simulink model "Control_Robot"  (R2018a)
settings: Solver=FixedStepAuto  StartTime=0.0  StopTime=10.0  FixedStep=0.01  RelTol=1e-3
undefined symbols (not defined in the file or in its folder): sigbuilder_block
libraries: simulink x2
settings Model: Creator=Amin  LastModifiedBy=Amin

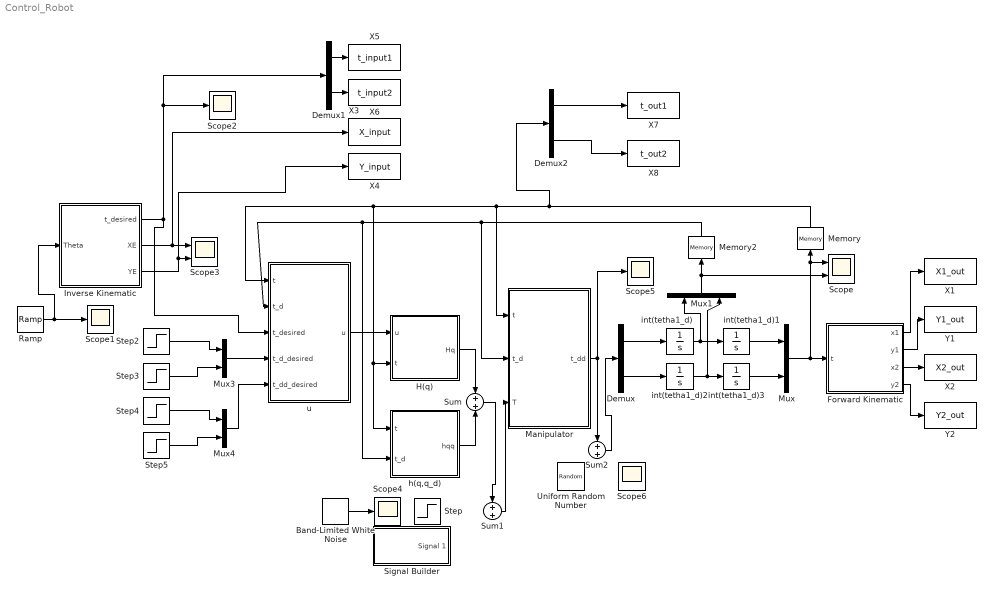
== system Control_Robot ==
   int(tetha1_d){,1..3} (4 alike) : Integrator
  Band-Limited White Noise : simulink/Sources/Band-Limited White Noise  Cov=[0.05]  Ts=0.1  seed=[23341]
  Demux : Demux  Outputs=2
  Demux1 : Demux  Outputs=2
  Demux2 : Demux  Outputs=2
  Forward Kinematic : MATLAB Function  TreatAsAtomicUnit=on
  H(q) : MATLAB Function  TreatAsAtomicUnit=on
  Inverse Kinematic : MATLAB Function  TreatAsAtomicUnit=on
  Manipulator : MATLAB Function  TreatAsAtomicUnit=on
  Memory : Memory  InitialCondition=[0 0]
  Memory2 : Memory  InitialCondition=[0 0]
  Mux{,1,3..4} (4 alike) : Mux  Inputs=2
  Ramp : simulink/Sources/Ramp  slope=1  start=1  InitialOutput=0
  Scope : Scope  NumInputPorts=2
  Scope{1..2,4..6} (5 alike) : Scope
  Scope3 : Scope  NumInputPorts=2
  Signal Builder : Subsystem  Tag=STV Subsys  LoadFcn=sigbuilder_block('load');  StartFcn=sigbuilder_block('start');  StopFcn=sigbuilder_block('stop');  ClipboardFcn=sigbuilder_block('clipboard');  mask(Sigbuilder block){tuvar=[0:10]}
      mask help: Simulink:masks:SigbuilderBlock_MD
      mask init:
      | if ~strcmp(get_param(bdroot(gcbh),'SimulationStatus'),'stopped') tuvar = sigbuilder_block('maskInit'); end
      settings: CopyFcn=sigbuilder_block('copy');  DeleteFcn=sigbuilder_block('delete');  ModelCloseFcn=sigbuilder_block('modelClose');  PreSaveFcn=sigbuilder_block('preSave');  PauseFcn=sigbuilder_block('pause');  ContinueFcn=sigbuilder_block('continue');  NameChangeFcn=sigbuilder_block('namechange');  OpenFcn=sigbuilder_block('open',[93 131.25 550.5 359.25 ]);  CloseFcn=sigbuilder_block('close');
      mask Display: plot(0, 0, 100, 100,[2, 2, 32, 32, 2], [68, 8, 8, 68, 68],[32, 2], [38, 38], [32, 19, 2],[53, 60, 44], [32, 17, 17, 2],[16, 16, 31, 31]);txt = getActiveGroup(gcbh);text(2, 100, txt,'verticalAlignment', 'top');
  Step : Step  After=6  SampleTime=0
  Step2 : Step  Before=0.01  After=0.01  SampleTime=0
  Step3 : Step  Before=0.01  After=0.01  SampleTime=0
  Step4 : Step  Before=0.001  After=0.001  SampleTime=0
  Step5 : Step  Before=0.001  After=0.001  SampleTime=0
  Sum : Sum  Inputs=+|+
  Sum1 : Sum  Inputs=+|+
  Sum2 : Sum  Inputs=+|+
  Uniform Random Number : UniformRandomNumber  Minimum=-3  Maximum=3  SampleTime=0.1
  X1 : ToWorkspace  VariableName=X1_out  SaveFormat=Structure With Time  SampleTime=-1
  X2 : ToWorkspace  VariableName=X2_out  SaveFormat=Structure With Time  SampleTime=-1
  X3 : ToWorkspace  VariableName=X_input  SaveFormat=Structure With Time  SampleTime=-1
  X4 : ToWorkspace  VariableName=Y_input  SaveFormat=Structure With Time  SampleTime=-1
  X5 : ToWorkspace  VariableName=t_input1  SaveFormat=Structure With Time  SampleTime=-1
  X6 : ToWorkspace  VariableName=t_input2  SaveFormat=Structure With Time  SampleTime=-1
  X7 : ToWorkspace  VariableName=t_out1  SaveFormat=Structure With Time  SampleTime=-1
  X8 : ToWorkspace  VariableName=t_out2  SaveFormat=Structure With Time  SampleTime=-1
  Y1 : ToWorkspace  VariableName=Y1_out  SaveFormat=Structure With Time  SampleTime=-1
  Y2 : ToWorkspace  VariableName=Y2_out  SaveFormat=Structure With Time  SampleTime=-1
  h(q,q_d) : MATLAB Function  TreatAsAtomicUnit=on
  u : MATLAB Function  TreatAsAtomicUnit=on
  wires:
  " int(tetha1_d)"/1 -> Mux1/1, " int(tetha1_d)1"/1
  " int(tetha1_d)2"/1 -> Mux1/2, " int(tetha1_d)3"/1
  Demux/1 -> " int(tetha1_d)"/1
  Demux/2 -> " int(tetha1_d)2"/1
  " int(tetha1_d)3"/1 -> Mux/2
  Mux/1 -> Scope/1, Memory/1, Forward Kinematic/1(t)
  Mux1/1 -> Scope/2, Memory2/1
  H(q)/1(Hq) -> Sum/1
  h(q,q_d)/1(hqq) -> Sum/2
  Memory2/1 -> Manipulator/2(t_d), u/2(t_d), h(q,q_d)/2(t_d)
  Memory/1 -> Demux2/1, u/1(t), h(q,q_d)/1(t), H(q)/2(t), Manipulator/1(t)
  u/1(u) -> H(q)/1(u)
  Forward Kinematic/1(x1) -> X1/1
  Forward Kinematic/2(y1) -> Y1/1
  Forward Kinematic/3(x2) -> X2/1
  Forward Kinematic/4(y2) -> Y2/1
  Step3/1 -> Mux3/2
  Step2/1 -> Mux3/1
  Step4/1 -> Mux4/1
  Step5/1 -> Mux4/2
  Mux4/1 -> u/5(t_dd_desired)
  Inverse Kinematic/1(t_desired) -> Demux1/1, Scope2/1, u/3(t_desired)
  Inverse Kinematic/2(XE) -> X3/1, Scope3/1
  Inverse Kinematic/3(YE) -> X4/1, Scope3/2
  Demux1/1 -> X5/1
  Demux1/2 -> X6/1
  Demux2/1 -> X7/1
  Demux2/2 -> X8/1
  Ramp/1 -> Scope1/1, Inverse Kinematic/1(Theta)
  Mux3/1 -> u/4(t_d_desired)
  " int(tetha1_d)1"/1 -> Mux/1
  Band-Limited White Noise/1 -> Scope4/1
  Manipulator/1(t_dd) -> Scope5/1, Sum2/1
  Sum2/1 -> Demux/1
  Sum/1 -> Sum1/1
  Sum1/1 -> Manipulator/3(T)

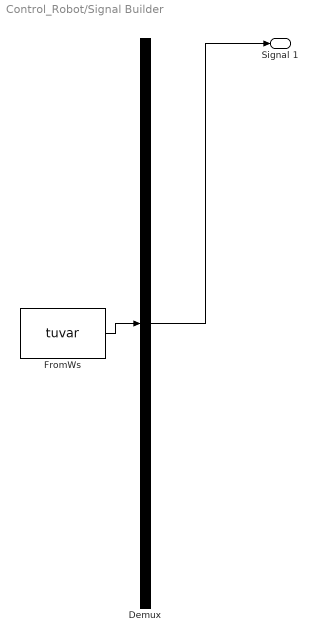
== system Control_Robot/Signal Builder ==
  Demux : Demux  Tag=STV Demux  Outputs=1
  FromWs : FromWorkspace  Tag=STV FromWs  VariableName=tuvar  SampleTime=0
      SigBuilderData=|
      | common.afterFinalStr = 'Extrapolate'
      | common.sampleTime = 0
      | dataSet.timeRange = [0 10]
      | dataSet.name = 'Group 1'
      | sbobj.Groups.Name = 'Group 1'
      | sbobj.Groups.Signals.Name = 'Signal 1'
      | sbobj.Groups.Signals.XData = [0 2.98 3 3 7 7 10]
      | sbobj.Groups.Signals.YData = [0 0 8 10 10 0 0]
  Signal 1 : Outport  Tag=STV Outport
  wires:
  Demux/1 -> Signal 1/1
  FromWs/1 -> Demux/1

== matlab function Control_Robot/H(q) ==
  data: u input; Hq output; t input
function Hq = fcn(u, t)
m1 = 1;
m2 = 1;
l1 = 1;
lc1 = 0.5;
l2 = 1;
lc2 = 0.5;
g = 9.81;

H11 = m1*lc1^2 + l1 + m2*(l1^2+lc2^2+2*l1*lc2*cos(t(2)))+l2;
H22 = m2*lc2^2 + l2;
H12 = m2*l1*lc2*cos(t(2)) + m2*lc2^2 + l2;
H21 = m2*l1*lc2*cos(t(2)) + m2*lc2^2 + l2;

H = [H11 H12; H21 H22];

Hq = H*u;

== matlab function Control_Robot/Manipulator ==
  data: t input; t_dd output; t_d input; T input
function t_dd = fcn(t, t_d, T)
m1 = 1;
m2 = 1;
l1 = 1;
lc1 = 0.5;
l2 = 1;
lc2 = 0.5;
g = 9.81;
H11 = m1*lc1^2 + l1 + m2*(l1^2+lc2^2+2*l1*lc2*cos(t(2)))+l2;
H22 = m2*lc2^2 + l2;
H12 = m2*l1*lc2*cos(t(2)) + m2*lc2^2 + l2;
H21 = m2*l1*lc2*cos(t(2)) + m2*lc2^2 + l2;
H = [H11 H12; H21 H22];
h = m2*l1*lc2*sin(t(2));
g1 = m1*lc1*g*cos(t(1)) + m2*g*(lc2*cos(t(1)+t(2))+l1*cos(t(1)));
g2 = m2*lc2*g*cos(t(1)+t(2));
t_dd = inv(H)*(T - [-h*t_d(2) -h*t_d(1)-h*t_d(2); h*t_d(1) 0]*[t_d(1); t_d(2)]-[g1; g2]);

== matlab function Control_Robot/h(q,q_d) ==
  data: t input; hqq output; t_d input
function hqq = fcn(t, t_d)

t1=t(1);
t2=t(2);
t_d1=t_d(1);
t_d2=t_d(2);

m1 = 1;
m2 = 1;
l1 = 1;
lc1 = 0.5;
l2 = 1;
lc2 = 0.5;
h = m2*l1*lc2*sin(t(2));
g = 9.81;

g1 = m1*lc1*g*cos(t1) + m2*g*(lc2*cos(t1+t2)+l1*cos(t1));
g2 = m2*lc2*g*cos(t1+t2);

hqq = [-h*t_d2 -h*t_d1-h*t_d2; h*t_d1 0]*[t_d1; t_d2]+[g1; g2];

== matlab function Control_Robot/Forward Kinematic ==
  data: t input; x1 output; y1 output; x2 output; y2 output

function [x1,y1,x2,y2] = fcn(t)
m1 = 1;
m2 = 1;
l1 = 1;
lc1 = 0.5;
l2 = 1;
lc2 = 0.5;
g = 9.81;
% Joint 2 location
x1 = l1*cos(t(1));
y1 = l1*sin(t(1));
% Joint 3 location
x2 = l1*cos(t(1))+l2*cos(t(1)+t(2));
y2 = l1*sin(t(1))+l2*sin(t(1)+t(2));

== matlab function Control_Robot/u ==
  data: t input; u output; t_d input; t_desired input; t_d_desired input; t_dd_desired input
function u = fcn(t, t_d, t_desired, t_d_desired, t_dd_desired)

KD = 20;
KP = 100;
tetha_tilted = t - t_desired;
tetha_d_tilted = t_d - t_d_desired;
u = t_dd_desired-(KD*(tetha_d_tilted))-(KP*(tetha_tilted));

== matlab function Control_Robot/Inverse Kinematic ==
  data: t_desired output; Theta input; XE output; YE output
function [t_desired, XE, YE] = fcn(Theta)
l1 = 1;
l2 = 1;
% Trajectory Design (Circle)
XE = 0.8 + 0.6*cos(Theta);
YE = 0.8 + 0.6*sin(Theta);
if Theta >= 2*3.14-0.2 && Theta <= 2*3.14+0.2
    XE = 1.4;
    YE = 0.8;
end

if Theta > 2*3.14+0.2
    XE = 2;
    YE = 0;
end

%% Trajectory 2
% r = Theta/10;
% XE = 0.8+ r*cos(Theta);
% YE = 0.8+ r*sin(Theta);

%% Inverse Kinematic
t1_desired =  2*atan((2*YE*l1 + (- XE^4 - 2*XE^2*YE^2 + 2*XE^2*l1^2 + 2*XE^2*l2^2 - YE^4 + 2*YE^2*l1^2 + 2*YE^2*l2^2 - l1^4 + 2*l1^2*l2^2 - l2^4)^(1/2))/(XE^2 + 2*XE*l1 + YE^2 + l1^2 - l2^2)); 
t2_desired =  2*atan((2*YE*l1 - (- XE^4 - 2*XE^2*YE^2 + 2*XE^2*l1^2 + 2*XE^2*l2^2 - YE^4 + 2*YE^2*l1^2 + 2*YE^2*l2^2 - l1^4 + 2*l1^2*l2^2 - l2^4)^(1/2))/(XE^2 + 2*XE*l1 + YE^2 + l1^2 - l2^2));
% Output Theta
t_desired = [t1_desired; t2_desired-t1_desired];
